simulink model "simulation_of_controlled_plant"  (R2020b)
settings: Solver=ode45  StartTime=0.0  StopTime=3  FixedStep=h  MaxStep=100  RelTol=1e-9  AbsTol=1e-9  EnableMultiTasking=on
Description:
  | Simulink Model for Pendubot by Leonid Freidovich
settings Model: Creator=Leonid Freidovich  LastModifiedBy=dell
settings SolverCC: AutoScaleAbsTol=off
settings DataIOCC: LimitDataPoints=on  SaveFormat=Array  SignalLoggingSaveFormat=ModelDataLogs  ReturnWorkspaceOutputs=off
settings OptimizationCC: BlockReduction=off  OptimizeBlockIOStorage=off  BufferReuse=off  GlobalBufferReuse=off  ExpressionFolding=off  ExpressionDepthLimit=2147483647  LocalBlockOutputs=off  InitFltsAndDblsToZero=on  LifeSpan=inf  OptimizeDataStoreBuffers=off  BusAssignmentInplaceUpdate=off
settings DebuggingCC: SaveWithParameterizedLinksMsg=none  UnderspecifiedInitializationDetection=Classic  MergeDetectMultiDrivingBlocksExec=none  SignalResolutionControl=TryResolveAllWithWarning  SolverPrmCheckMsg=warning  MultiTaskDSMMsg=warning  MultiTaskCondExecSysMsg=none  FcnCallInpInsideContextMsg=warning  StateNameClashWarn=warning  SFUnexpectedBacktrackingDiag=warning  SFNoUnconditionalDefaultTransitionDiag=warning  SFExecutionAtInitializationDiag=none  ArithmeticOperatorsInVariantConditions=warning
settings HardwareCC: ProdBitPerPointer=32  ProdBitPerSizeT=32  ProdBitPerPtrDiffT=32  ProdLargestAtomicFloat=None  ProdEndianess=BigEndian  ProdWordSize=32  ProdHWDeviceType=Specified  TargetHWDeviceType=32-bit Generic  ProdEqTarget=off
settings ModelReferenceCC: PropagateSignalLabelsOutOfModel=off
settings SFSimCC: SimUseLocalCustomCode=off  CustomCodeUndefinedFunction=UseInterfaceOnly
settings RTWCC: Description="Visual C/C++ Project Makefile only for the \"grt\" target"  GenerateMakefile=off  TemplateMakefile=grt_msvc.tmf  RTWUseLocalCustomCode=off  RTWCompilerOptimization=on
settings CodeAppCC: StateflowObjectComments=on
settings GRTTargetCC: TargetLangStandard=C89/C90 (ANSI)  CombineOutputUpdateFcns=off  GRTInterface=on  UseToolchainInfoCompliant=off
settings ConfigComp: CovMetricSettings=dw  CovSaveCumulativeToWorkspaceVar=on  CovSaveSingleToWorkspaceVar=on  CovExternalEMLEnable=off

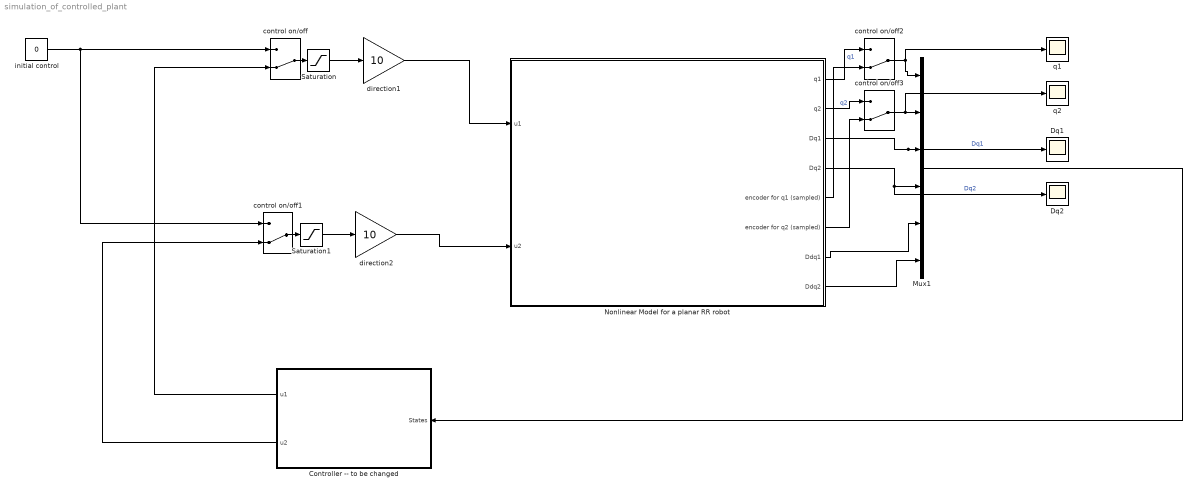
== system simulation_of_controlled_plant ==
  "Controller -- to be changed" : Subsystem
  Dq1 : Scope
  Dq2 : Scope
  Mux1 : Mux  Inputs=6
  Nonlinear Model for a planar RR robot : Subsystem
  Saturation : Saturate  UpperLimit=10  LowerLimit=-10
  Saturation1 : Saturate  UpperLimit=10  LowerLimit=-10
  control on/off{,1..3} (4 alike) : ManualSwitch  CurrentSetting=0
  direction1 : Gain  Gain=10  SaturateOnIntegerOverflow=on  OutDataTypeStr=Inherit: Same as input  ParamDataTypeStr=Inherit: Same as input
  direction2 : Gain  Gain=10  SaturateOnIntegerOverflow=on  OutDataTypeStr=Inherit: Same as input  ParamDataTypeStr=Inherit: Same as input
  initial control : Constant  Value=0
  q1 : Scope
  q2 : Scope
  wires:
  Saturation/1 -> direction1/1
  control on/off/1 -> Saturation/1
  initial control/1 -> control on/off1/1, control on/off/1
  direction1/1 -> Nonlinear Model for a planar RR robot/1(u1)
  Nonlinear Model for a planar RR robot/3(Dq1) -> Dq1/1, Mux1/3  "Dq1"
  Nonlinear Model for a planar RR robot/4(Dq2) -> Dq2/1, Mux1/4  "Dq2"
  Mux1/1 -> "Controller -- to be changed"/1(States)
  control on/off1/1 -> Saturation1/1
  Saturation1/1 -> direction2/1
  direction2/1 -> Nonlinear Model for a planar RR robot/2(u2)
  "Controller -- to be changed"/2(u2) -> control on/off1/2
  "Controller -- to be changed"/1(u1) -> control on/off/2
  Nonlinear Model for a planar RR robot/7(Ddq1) -> Mux1/5
  Nonlinear Model for a planar RR robot/8(Ddq2) -> Mux1/6
  Nonlinear Model for a planar RR robot/5(encoder for q1 (sampled)) -> control on/off2/2
  Nonlinear Model for a planar RR robot/6(encoder for q2 (sampled)) -> control on/off3/2
  Nonlinear Model for a planar RR robot/1(q1) -> control on/off2/1  "q1"
  control on/off2/1 -> Mux1/1, q1/1
  control on/off3/1 -> q2/1, Mux1/2
  Nonlinear Model for a planar RR robot/2(q2) -> control on/off3/1  "q2"

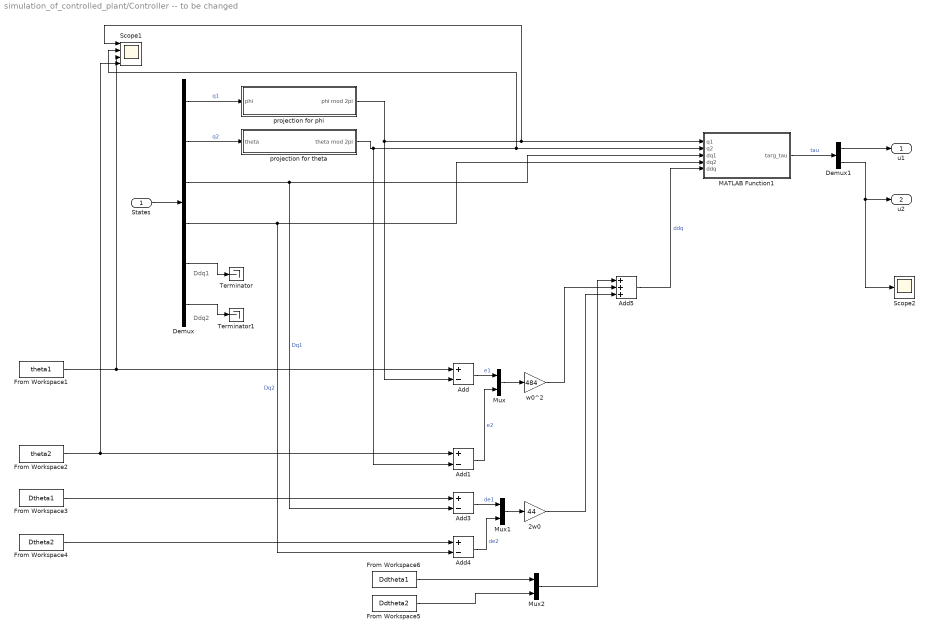
== system simulation_of_controlled_plant/Controller -- to be changed ==
  note: Ddq2
  note: Ddq1
  States : Inport
  2w0 : Gain  Gain=44
  Add{,1,3..4} (4 alike) : Sum  Inputs=+-
  Add5 : Sum  Inputs=+++
  Demux : Demux  Outputs=6
      settings: DisplayOption=none
  Demux1 : Demux  Outputs=2
  From Workspace1 : FromWorkspace  VariableName=theta1
  From Workspace2 : FromWorkspace  VariableName=theta2
  From Workspace3 : FromWorkspace  VariableName=Dtheta1
  From Workspace4 : FromWorkspace  VariableName=Dtheta2
  From Workspace5 : FromWorkspace  VariableName=Ddtheta2
  From Workspace6 : FromWorkspace  VariableName=Ddtheta1
  MATLAB Function1 : MATLAB Function  TreatAsAtomicUnit=on
  Mux : Mux  Inputs=2
  Mux1 : Mux  Inputs=2
  Mux2 : Mux  Inputs=2
  Scope1 : Scope  NumInputPorts=4
  Scope2 : Scope
  Terminator : Terminator
  Terminator1 : Terminator
  projection for phi : Subsystem
  projection for theta : Subsystem
  w0^2 : Gain  Gain=484
  u1 : Outport  VectorParamsAs1DForOutWhenUnconnected=off
  u2 : Outport  Port=2  VectorParamsAs1DForOutWhenUnconnected=off
  wires:
  States/1 -> Demux/1
  Demux/1 -> projection for phi/1(phi)  "q1"
  Demux/2 -> projection for theta/1(theta)  "q2"
  Demux1/1 -> u1/1
  Demux1/2 -> Scope2/1, u2/1
  From Workspace1/1 -> Scope1/3, Add/1
  From Workspace2/1 -> Add1/1, Scope1/4
  Add/1 -> Mux/1  "e1"
  Add1/1 -> Mux/2  "e2"
  Mux/1 -> w0^2/1
  Demux/3 -> Add3/2, MATLAB Function1/3(dq1)  "Dq1"
  Demux/4 -> Add4/2, MATLAB Function1/4(dq2)  "Dq2"
  Add3/1 -> Mux1/1  "de1"
  Add4/1 -> Mux1/2  "de2"
  Mux1/1 -> 2w0/1
  Mux2/1 -> Add5/1
  2w0/1 -> Add5/3
  w0^2/1 -> Add5/2
  Demux/5 -> Terminator/1
  Demux/6 -> Terminator1/1
  Add5/1 -> MATLAB Function1/5(ddq)  "ddq"
  projection for phi/1(phi mod 2pi) -> Scope1/1, MATLAB Function1/1(q1), Add/2
  From Workspace3/1 -> Add3/1
  From Workspace4/1 -> Add4/1
  From Workspace5/1 -> Mux2/2
  From Workspace6/1 -> Mux2/1
  MATLAB Function1/1(targ_tau) -> Demux1/1  "tau"
  projection for theta/1(theta mod 2pi) -> Add1/2, Scope1/2, MATLAB Function1/2(q2)

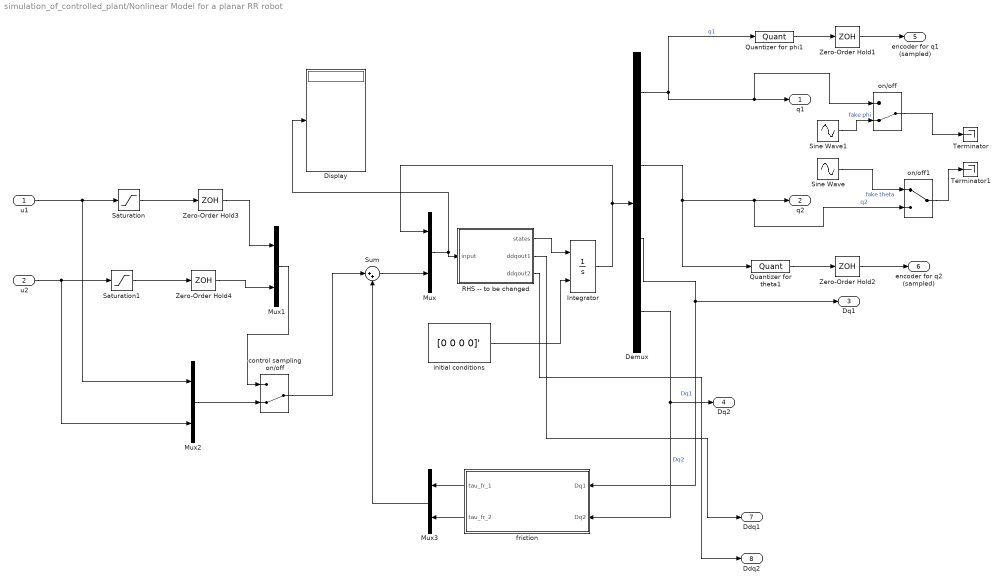
== system simulation_of_controlled_plant/Nonlinear Model for a planar RR robot ==
  u1 : Inport
  u2 : Inport  Port=2
  Demux : Demux
      settings: DisplayOption=none
  Display : Display
  Integrator : Integrator  InitialConditionSource=external  InitialCondition=[-pi/2 0 0 0]
  Mux{,1..3} (4 alike) : Mux  Inputs=2
  Quantizer for phi1 : Quantizer  QuantizationInterval=2*pi/1024/4
  Quantizer for theta1 : Quantizer  QuantizationInterval=2*pi/1024/4
  "RHS -- to be changed" : Subsystem
  Saturation : Saturate  UpperLimit=10  LowerLimit=-10
  Saturation1 : Saturate  UpperLimit=10  LowerLimit=-10
  Sine Wave : Sin  Amplitude=3  Frequency=0.4  SampleTime=0
  Sine Wave1 : Sin  Amplitude=3  Frequency=0.4  SampleTime=0
  Sum : Sum  Inputs=|++  SaturateOnIntegerOverflow=on
  Terminator : Terminator
  Terminator1 : Terminator
  Zero-Order Hold{1..4} (4 alike) : ZeroOrderHold  SampleTime=0.001
  control sampling on/off : ManualSwitch  CurrentSetting=0
  friction : Subsystem
  initial conditions : Constant  Value=[0 0 0 0]'
  on/off : ManualSwitch  CurrentSetting=0
  on/off1 : ManualSwitch
  q1 : Outport  VectorParamsAs1DForOutWhenUnconnected=off
  q2 : Outport  Port=2  VectorParamsAs1DForOutWhenUnconnected=off
  Dq1 : Outport  Port=3  VectorParamsAs1DForOutWhenUnconnected=off
  Dq2 : Outport  Port=4  VectorParamsAs1DForOutWhenUnconnected=off
  encoder for q1 (sampled) : Outport  Port=5  VectorParamsAs1DForOutWhenUnconnected=off
  encoder for q2 (sampled) : Outport  Port=6  VectorParamsAs1DForOutWhenUnconnected=off
  Ddq1 : Outport  Port=7  VectorParamsAs1DForOutWhenUnconnected=off
  Ddq2 : Outport  Port=8  VectorParamsAs1DForOutWhenUnconnected=off
  wires:
  Mux/1 -> Display/1, "RHS -- to be changed"/1(input)
  Integrator/1 -> Demux/1, Mux/1
  Demux/1 -> on/off/1, q1/1, Quantizer for phi1/1  "q1"
  Demux/2 -> Quantizer for theta1/1, on/off1/2, q2/1  "q2"
  Demux/3 -> friction/1(Dq1), Dq1/1  "Dq1"
  Demux/4 -> friction/2(Dq2), Dq2/1  "Dq2"
  Quantizer for phi1/1 -> Zero-Order Hold1/1
  Zero-Order Hold1/1 -> encoder for q1 (sampled)/1
  Quantizer for theta1/1 -> Zero-Order Hold2/1
  Zero-Order Hold2/1 -> encoder for q2 (sampled)/1
  Sum/1 -> Mux/2
  Saturation/1 -> Zero-Order Hold3/1
  u1/1 -> Mux2/1, Saturation/1
  u2/1 -> Mux2/2, Saturation1/1
  Saturation1/1 -> Zero-Order Hold4/1
  Zero-Order Hold3/1 -> Mux1/1
  Zero-Order Hold4/1 -> Mux1/2
  Mux2/1 -> control sampling on/off/2
  Mux1/1 -> control sampling on/off/1
  control sampling on/off/1 -> Sum/1
  initial conditions/1 -> Integrator/2
  friction/1(tau_fr_1) -> Mux3/1
  friction/2(tau_fr_2) -> Mux3/2
  Mux3/1 -> Sum/2
  Sine Wave1/1 -> on/off/2  "fake phi"
  on/off/1 -> Terminator/1
  Sine Wave/1 -> on/off1/1  "fake theta"
  on/off1/1 -> Terminator1/1
  "RHS -- to be changed"/1(states) -> Integrator/1
  "RHS -- to be changed"/2(ddqout1) -> Ddq1/1
  "RHS -- to be changed"/3(ddqout2) -> Ddq2/1

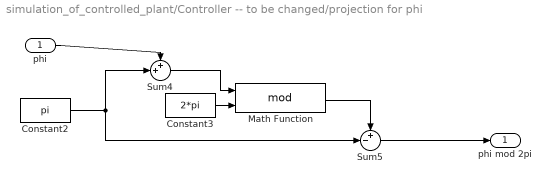
== system simulation_of_controlled_plant/Controller -- to be changed/projection for phi ==
  phi : Inport
  Constant2 : Constant  Value=pi
  Constant3 : Constant  Value=2*pi
  Math Function : Math  Operator=mod  SignedPower=on  SaturateOnIntegerOverflow=on
  Sum4 : Sum  Inputs=++|
  Sum5 : Sum  Inputs=+-|
  phi mod 2pi : Outport  VectorParamsAs1DForOutWhenUnconnected=off
  wires:
  phi/1 -> Sum4/1
  Sum5/1 -> phi mod 2pi/1
  Math Function/1 -> Sum5/1
  Constant3/1 -> Math Function/2
  Sum4/1 -> Math Function/1
  Constant2/1 -> Sum5/2, Sum4/2

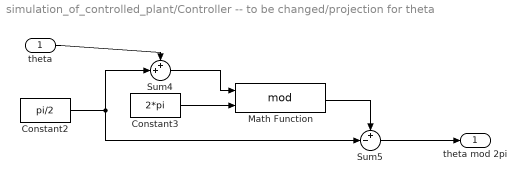
== system simulation_of_controlled_plant/Controller -- to be changed/projection for theta ==
  theta : Inport
  Constant2 : Constant  Value=pi/2
  Constant3 : Constant  Value=2*pi
  Math Function : Math  Operator=mod  SignedPower=on  SaturateOnIntegerOverflow=on
  Sum4 : Sum  Inputs=++|
  Sum5 : Sum  Inputs=+-|
  theta mod 2pi : Outport  VectorParamsAs1DForOutWhenUnconnected=off
  wires:
  theta/1 -> Sum4/1
  Sum5/1 -> theta mod 2pi/1
  Math Function/1 -> Sum5/1
  Constant3/1 -> Math Function/2
  Sum4/1 -> Math Function/1
  Constant2/1 -> Sum5/2, Sum4/2

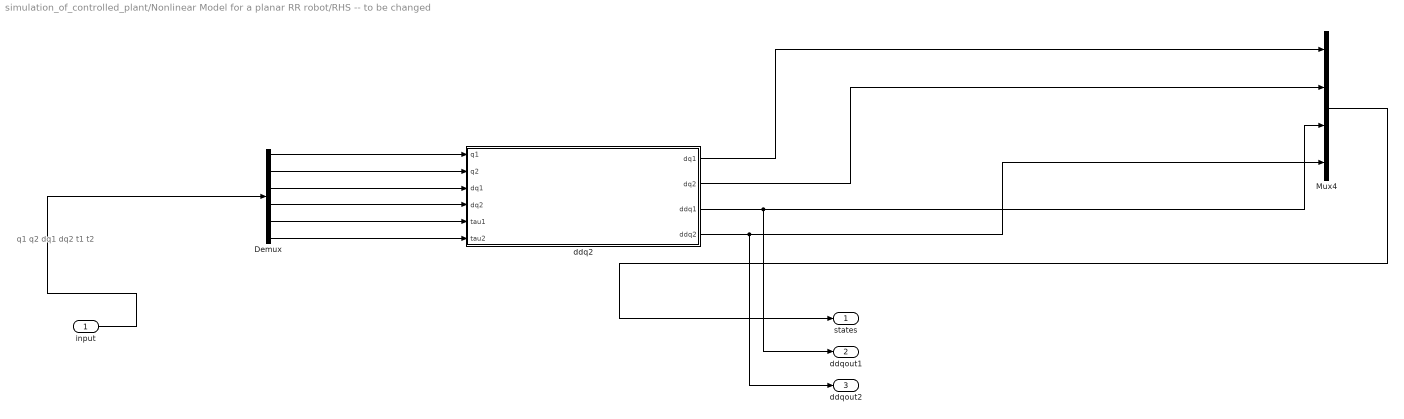
== system simulation_of_controlled_plant/Nonlinear Model for a planar RR robot/RHS -- to be changed ==
  note: q1
      | q2
      | dq1
      | dq2
      | t1
      | t2
  input : Inport
  Demux : Demux  Outputs=6
  Mux4 : Mux
  ddq2 : MATLAB Function  TreatAsAtomicUnit=on
  states : Outport  VectorParamsAs1DForOutWhenUnconnected=off
  ddqout1 : Outport  Port=2  VectorParamsAs1DForOutWhenUnconnected=off
  ddqout2 : Outport  Port=3  VectorParamsAs1DForOutWhenUnconnected=off
  wires:
  ddq2/3(ddq1) -> ddqout1/1, Mux4/3
  input/1 -> Demux/1
  Mux4/1 -> states/1
  Demux/1 -> ddq2/1(q1)
  Demux/2 -> ddq2/2(q2)
  ddq2/4(ddq2) -> ddqout2/1, Mux4/4
  ddq2/2(dq2) -> Mux4/2
  ddq2/1(dq1) -> Mux4/1
  Demux/3 -> ddq2/3("dq1 ")
  Demux/4 -> ddq2/4("dq2 ")
  Demux/5 -> ddq2/5(tau1)
  Demux/6 -> ddq2/6(tau2)

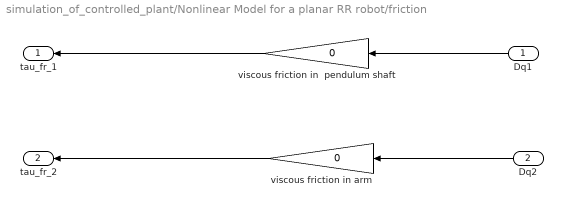
== system simulation_of_controlled_plant/Nonlinear Model for a planar RR robot/friction ==
  Dq1 : Inport
  Dq2 : Inport  Port=2
  viscous friction in  pendulum shaft : Gain  Gain=0  SaturateOnIntegerOverflow=on  OutDataTypeStr=Inherit: Same as input  ParamDataTypeStr=Inherit: Same as input
  viscous friction in arm : Gain  Gain=0  SaturateOnIntegerOverflow=on  OutDataTypeStr=Inherit: Same as input  ParamDataTypeStr=Inherit: Same as input
  tau_fr_1 : Outport  VectorParamsAs1DForOutWhenUnconnected=off
  tau_fr_2 : Outport  Port=2  VectorParamsAs1DForOutWhenUnconnected=off
  wires:
  Dq1/1 -> viscous friction in  pendulum shaft/1
  Dq2/1 -> viscous friction in arm/1
  viscous friction in  pendulum shaft/1 -> tau_fr_1/1
  viscous friction in arm/1 -> tau_fr_2/1

== matlab function simulation_of_controlled_plant/Nonlinear Model for a planar RR robot/RHS -- to be changed/ddq2 ==
  data: dq1 output; dq2 output; ddq1 output; ddq2 output; q1 input; q2 input; dq1 input; dq2 input; tau1 input; tau2 input
function [dq1, dq2, ddq1, ddq2] = fcn(q1,q2,dq1,dq2,tau1,tau2)

dq =[0,0];
dq(1)=dq1;
dq(2)=dq2;
ddq=[0,0];

g=9.81;
l1=0.25;
lc1=0.198;
lc2=0.109;
m1=0.374;
m2=0.129;
I1=0.0027;
I2=0.00113;

G =[g*cos(q1)*(l1*m2 + lc1*m1) + g*lc2*m2*cos(q1 + q2);g*lc2*m2*cos(q1 + q2)];

M =[m2*l1^2 + 2*m2*cos(q2)*l1*lc2 + m1*lc1^2 + m2*lc2^2 + I1 + I2, m2*lc2^2 + l1*m2*cos(q2)*lc2 + I2; 
    m2*lc2^2 + l1*m2*cos(q2)*lc2 + I2, m2*lc2^2 + I2];
 
C =[-dq(2)*l1*lc2*m2*sin(q2), - dq(1)*l1*lc2*m2*sin(q2) - dq(2)*l1*lc2*m2*sin(q2);
    -dq(1)*l1*lc2*m2*sin(q2),                                               0];

ddq=inv(M)*(-C*[dq(1) dq(2)]'-G+[tau1 tau2]');

ddq1=ddq(1);
ddq2=ddq(2);

== matlab function simulation_of_controlled_plant/Controller -- to be changed/MATLAB Function1 ==
  data: q1 input; targ_tau output; q2 input; dq1 input; dq2 input; ddq input
function targ_tau = fcn(q1, q2, dq1, dq2, ddq)
 
ddq1=ddq(1); ddq2=ddq(2);
g=9.81;
l1=0.25;
lc1=0.198;
lc2=0.109;
m1=0.374;
m2=0.129;
I1=0.0027;
I2=0.00113;

G =[g*cos(q1)*(l1*m2 + lc1*m1) + g*lc2*m2*cos(q1 + q2);g*lc2*m2*cos(q1 + q2)];

M =[m2*l1^2 + 2*m2*cos(q2)*l1*lc2 + m1*lc1^2 + m2*lc2^2 + I1 + I2, m2*lc2^2 + l1*m2*cos(q2)*lc2 + I2; 
    m2*lc2^2 + l1*m2*cos(q2)*lc2 + I2, m2*lc2^2 + I2];
 
C =[-dq2*l1*lc2*m2*sin(q2), - dq1*l1*lc2*m2*sin(q2) - dq2*l1*lc2*m2*sin(q2);
    -dq1*l1*lc2*m2*sin(q2),                                               0];

ddq=[ddq1;ddq2];
dq=[dq1;dq2];
tau_matrix = M*ddq+G+C*dq;

tau1=tau_matrix(1,1);
tau2=tau_matrix(2,1);

%output
targ_tau = [tau1,tau2];
